simulink model "Main_Sims"  (R2019b)
settings: Solver=ode45  StartTime=0.0  StopTime=10  RelTol=1e-3  EnableMultiTasking=on
values from neighbouring files (symbols this model uses):
  A = [0, 0, 1, 0; 0, 0, 0, 1; 0, 0, 0, 0; 0, 0, 0, 0]    [Main_Code.m]
  B = [0; 0; 0; 0]    [Main_Code.m]
  C = eye(4)    [Main_Code.m]
  D = [0; 0; 0; 0]    [Main_Code.m]
  K = lqr(A, B, Q, R)    [Main_Code.m]
settings Model: Creator=CCLab  LastModifiedBy=CCLab
settings DataIOCC: LimitDataPoints=on  SaveFormat=Array  ReturnWorkspaceOutputs=off
settings OptimizationCC: LifeSpan=inf
settings DebuggingCC: SolverPrmCheckMsg=warning  SFUnexpectedBacktrackingDiag=warning  SFNoUnconditionalDefaultTransitionDiag=warning  SFExecutionAtInitializationDiag=none  ArithmeticOperatorsInVariantConditions=warning
settings HardwareCC: ProdBitPerPointer=32  ProdBitPerSizeT=32  ProdBitPerPtrDiffT=32  ProdLargestAtomicFloat=None  ProdIntDivRoundTo=Undefined  ProdEndianess=Unspecified  ProdWordSize=32  ProdHWDeviceType=32-bit Generic
settings ModelReferenceCC: PropagateSignalLabelsOutOfModel=off
settings SFSimCC: SimUseLocalCustomCode=off  CustomCodeUndefinedFunction=UseInterfaceOnly
settings RTWCC: RTWUseLocalCustomCode=off
settings CodeAppCC: StateflowObjectComments=on
settings GRTTargetCC: TargetLangStandard=C89/C90 (ANSI)  GeneratePreprocessorConditionals=Disable all
settings ConfigComp: CovMetricSettings=dw  CovHtmlReporting=on  CovSaveCumulativeToWorkspaceVar=on  CovSaveSingleToWorkspaceVar=on  CovExternalEMLEnable=off  CovSFcnEnable=off

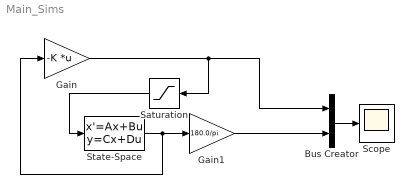
== system Main_Sims ==
  Bus Creator : BusCreator  Inputs=2
  Gain : Gain  Gain=-K  Multiplication=Matrix(K*u)
  Gain1 : Gain  Gain=180.0/pi
  Saturation : Saturate  UpperLimit=12  LowerLimit=-12
  Scope : Scope
  State-Space : StateSpace  A=A  B=B  C=C  D=D  InitialCondition=[pi/12 3/180*pi 0 0]
  wires:
  Bus Creator/1 -> Scope/1
  Gain1/1 -> Bus Creator/2
  State-Space/1 -> Gain/1, Gain1/1
  Gain/1 -> Saturation/1, Bus Creator/1
  Saturation/1 -> State-Space/1
